simulink subsystem "AdasCorePlantModel"  (R2023a)
settings: Solver=VariableStepAuto  StartTime=0.0  StopTime=10.0  RelTol=1e-3
undefined symbols (not defined in the file or in its folder): BalNotActWait, BalOffWait, BalOnWait, Battery, contactorTime, CtrlBcuTrlrBrkGain, CtrlTcuInitGear, CtrlVcuCltch1InitCmd, CtrlVcuEvChrgLmtBpt, CtrlVcuEvRegenBrkCutOff, CtrlVcuEvRegenBrkSpdBpt, CtrlVcuEvSocBpt, currentFactor, CV_Gain, DiscIntNeverNeededParam, EnvAbsPrs, EnvAirTemp, EnvNomFrictionScaling, EnvNominalGrade, EnvWindVelX, EnvWindVelY, EnvWindVelZ, flgEnBalancing, HighTempLimit, I_cc, LowTempLimit, MaxCellVoltThrsld, MaxChrgCurrLim, MaxDchrgCurrLim, MinCellVoltDchrgCurrentLim_BP, MinCellVoltDchrgCurrentLim_Table, noCurrent, OverCellVoltageLimit, PlntBattModNumCellPar, PlntBattModNumCellSer, PlntBattNumMod, PlntBattSocInit, PlntBattTempInitDegC, PlntBrkActrBoreFrnt, PlntBrkFrntBias, PlntBrkKinFricCffFrnt, PlntBrkNumPadsFrnt, PlntBrkPadMeanRadiusFrnt, PlntBrkPrsFctr, PlntBrkRearBias, PlntDiffrntlRatio, PlntEM1EffTbl, PlntEM1Spd, PlntEM1Trq, PlntEM1TrqEff, PlntVehDstCGFrntAxl, PlntVehDstCGRearAxl, SnsrFltThld, TargetDeltaV, timeoutContactor, timeoutCurrent, Ts, UnderCellVoltageLimit, voltThreshold, vRatio
libraries: simulink x10, sharedTrackingLibrary x2, autolibutils x1
(part 3 of 4)

== system AdasCorePlantModel/Controllers/Vehicle Control Unit (VCU)/EV 1EM with BMS (non-reference)/Power Limit Calculations ==
  note: Use Current Limits from BMS to calculate
      | discharge and charge power limits
  PackVolt : Inport
  BMSDischrgCurrLmt : Inport  Port=2
  BMSChrgCurrLmt : Inport  Port=3
  Data Type Conversion : DataTypeConversion  SaturateOnIntegerOverflow=off  RndMeth=Floor
  Data Type Conversion1 : DataTypeConversion  SaturateOnIntegerOverflow=off  RndMeth=Floor
  Gain : Gain  Gain=-1
  Gain1 : Gain  Gain=-1
  Product : Product
  Product1 : Product
  BattPwrDischrgLmt : Outport  VectorParamsAs1DForOutWhenUnconnected=off
  BattPwrChrgLmt : Outport  Port=2  VectorParamsAs1DForOutWhenUnconnected=off
  wires:
  Data Type Conversion1/1 -> BattPwrDischrgLmt/1
  Data Type Conversion/1 -> BattPwrChrgLmt/1
  BMSDischrgCurrLmt/1 -> Gain1/1
  BMSChrgCurrLmt/1 -> Gain/1
  PackVolt/1 -> Product1/1, Product/1
  Product1/1 -> Data Type Conversion/1
  Product/1 -> Data Type Conversion1/1
  Gain1/1 -> Product/2
  Gain/1 -> Product1/2

== system AdasCorePlantModel/Controllers/Vehicle Control Unit (VCU)/EV 1EM with BMS (non-reference)/Regen Braking Control ==
  "BattSoc " : Inport
  "VehSpd " : Inport  Port=2
  "EMSpd " : Inport  Port=3
  "BrkPrsReq " : Inport  Port=4
  Parallel Regen Braking : Subsystem  InitFcn=[~]=autosharedicon('autolibinternalvvblock',gcb,0,'6');  VariantControl=(default)
  Series Regen Braking : Subsystem  InitFcn=%[~]=autosharedicon('autolibinternalvvblock',gcb,0,'6');  VariantControl=Variant
  " EMTrqCmdRegen" : Outport  VectorParamsAs1DForOutWhenUnconnected=off
  " BrkCmd" : Outport  Port=2  VectorParamsAs1DForOutWhenUnconnected=off

== system AdasCorePlantModel/Controllers/Vehicle Control Unit (VCU)/EV 1EM with BMS (non-reference)/Subsystem2 ==
  SOC : Inport
  Data Type Conversion : DataTypeConversion  SaturateOnIntegerOverflow=off  RndMeth=Floor
  convert2percent : Gain  Gain=100
  BattSOC : Outport
  wires:
  Data Type Conversion/1 -> BattSOC/1
  SOC/1 -> convert2percent/1
  convert2percent/1 -> Data Type Conversion/1

== system AdasCorePlantModel/Controllers/Vehicle Control Unit (VCU)/EV 1EM with BMS (non-reference)/Trailer Brake Pressure Command ==
  BrkCmd : Inport
  Gain1 : Gain  Gain=CtrlBcuTrlrBrkGain
  Probe : Probe  ProbeSampleTime=off  ProbeComplexSignal=off
  Product : Product  Inputs=*/
  Selector2 : Selector  InputPortWidth=1  IndexOptions=Index vector (dialog)  Indices=[1 1 1 1 1 1]  OutputSizes=1
  Sum : Sum  Inputs=+
  VcuTrlrBrkPrsCmd : Outport
  wires:
  Selector2/1 -> VcuTrlrBrkPrsCmd/1
  Sum/1 -> Product/1
  BrkCmd/1 -> Sum/1, Probe/1
  Probe/1 -> Product/2
  Product/1 -> Gain1/1
  Gain1/1 -> Selector2/1

== system AdasCorePlantModel/Environment/Varying Friction/Varying Friction/Road Track Friction ==
  XWhl : Inport
  YWhl : Inport  Port=2
  Cg : Inport  Port=3
  2D Lookup Tbl for Scaling Fctr (Lambda) : Subsystem  TreatAsAtomicUnit=on
      mask init:
      | [~]=vehdynicon('vehdynblk',gcb);
  Bus Selector : BusSelector  OutputSignals=X,Y
  Cnst Lambda : Constant  Value=ones(4,1).*lambda_g
  Constant1 : Constant  Value=SplitLambdaTrck
  Creating Inertial Frm Bpt : Subsystem
  En at t = 0 : Subsystem
  "Lambda (t = 0) " : Memory  InitialCondition=ones(4,1).*lambda_g  InheritSampleTime=on
  Switch : Switch  Criteria=u2 > Threshold  SaturateOnIntegerOverflow=off  InputSameDT=off
  FricCoeffLambda : Outport
  wires:
  YWhl/1 -> 2D Lookup Tbl for Scaling Fctr (Lambda)/2(YWhl)
  XWhl/1 -> 2D Lookup Tbl for Scaling Fctr (Lambda)/1(XWhl)
  2D Lookup Tbl for Scaling Fctr (Lambda)/1(Lambda for each whl) -> Switch/1
  "Lambda (t = 0) "/1 -> FricCoeffLambda/1
  Switch/1 -> "Lambda (t = 0) "/1
  Cnst Lambda/1 -> Switch/3
  Constant1/1 -> Switch/2
  Cg/1 -> Bus Selector/1
  Creating Inertial Frm Bpt/1(XBpt) -> 2D Lookup Tbl for Scaling Fctr (Lambda)/3(XBpt)
  Creating Inertial Frm Bpt/2(YBpt) -> 2D Lookup Tbl for Scaling Fctr (Lambda)/4(YBpt)
  Bus Selector/1 -> Creating Inertial Frm Bpt/1(XCg)  "<X>"
  Bus Selector/2 -> Creating Inertial Frm Bpt/2(YCg)  "<Y>"
  En at t = 0/1(Out1) -> Creating Inertial Frm Bpt/Enable

== system AdasCorePlantModel/Environment/Varying Friction/Varying Friction/Wheel Coordinates ==
  FrntAxlLftX : Inport
  FrntAxlRghtX : Inport  Port=2
  RearAxlLftX : Inport  Port=3
  RearAxlRghtX : Inport  Port=4
  FrntAxlLftY : Inport  Port=5
  FrntAxlRghtY : Inport  Port=6
  RearAxlLftY : Inport  Port=7
  RearAxlRghtY : Inport  Port=8
  Matrix Concatenate : Concatenate  NumInputs=4  Mode=Multidimensional array
  Matrix Concatenate1 : Concatenate  NumInputs=4  Mode=Multidimensional array
  XWhl : Outport
  YWhl : Outport  Port=2
  wires:
  RearAxlRghtX/1 -> Matrix Concatenate/4
  Matrix Concatenate/1 -> XWhl/1
  RearAxlRghtY/1 -> Matrix Concatenate1/4
  RearAxlLftX/1 -> Matrix Concatenate/3
  RearAxlLftY/1 -> Matrix Concatenate1/3
  FrntAxlRghtX/1 -> Matrix Concatenate/2
  FrntAxlRghtY/1 -> Matrix Concatenate1/2
  FrntAxlLftY/1 -> Matrix Concatenate1/1
  FrntAxlLftX/1 -> Matrix Concatenate/1
  Matrix Concatenate1/1 -> YWhl/1

== system AdasCorePlantModel/Vehicle/Trailer Input/Ground Info Trailer/Ground Info 2 AxleTrailer ==
  Env : Inport
  Bus Selector1 : BusSelector  OutputSignals=TraGnd.z.G_FL_z,TraGnd.z.G_FR_z,TraGnd.z.G_RL_z,TraGnd.z.G_RR_z
  Bus Selector3 : BusSelector  OutputSignals=Gnd.mu.mu_FL,Gnd.mu.mu_FR,Gnd.mu.mu_RL,Gnd.mu.mu_RR
  Vector Concatenate : Concatenate  NumInputs=4
  Vector Concatenate1 : Concatenate  NumInputs=4
  Ground : Outport
  Friction : Outport  Port=2
  wires:
  Bus Selector3/4 -> Vector Concatenate/4  "<mu_RR>"
  Bus Selector3/3 -> Vector Concatenate/3  "<mu_RL>"
  Bus Selector1/1 -> Vector Concatenate1/1  "<G_FL_z>"
  Bus Selector1/2 -> Vector Concatenate1/2  "<G_FR_z>"
  Bus Selector1/3 -> Vector Concatenate1/3  "<G_RL_z>"
  Bus Selector1/4 -> Vector Concatenate1/4  "<G_RR_z>"
  Bus Selector3/2 -> Vector Concatenate/2  "<mu_FR>"
  Bus Selector3/1 -> Vector Concatenate/1  "<mu_FL>"
  Vector Concatenate/1 -> Friction/1
  Vector Concatenate1/1 -> Ground/1
  Env/1 -> Bus Selector1/1, Bus Selector3/1

== system AdasCorePlantModel/Vehicle/Trailer Input/Ground Info Trailer/Ground Info 3 AxleTrailer ==
  Env : Inport
  Bus Selector1 : BusSelector  OutputSignals=TraGnd.z.G_FL_z,TraGnd.z.G_FR_z,TraGnd.z.G_RL_z,TraGnd.z.G_RR_z,TraGnd.z.G_RL_z,TraGnd.z.G_RR_z
  Bus Selector3 : BusSelector  OutputSignals=TraGnd.mu.mu_FL,TraGnd.mu.mu_FR,TraGnd.mu.mu_RL,TraGnd.mu.mu_RR,TraGnd.mu.mu_RL,TraGnd.mu.mu_RR
  Vector Concatenate : Concatenate  NumInputs=6
  Vector Concatenate1 : Concatenate  NumInputs=6
  Ground : Outport
  Friction : Outport  Port=2
  wires:
  Env/1 -> Bus Selector3/1, Bus Selector1/1
  Vector Concatenate1/1 -> Ground/1
  Vector Concatenate/1 -> Friction/1
  Bus Selector3/1 -> Vector Concatenate/1  "<mu_FL>"
  Bus Selector3/2 -> Vector Concatenate/2  "<mu_FR>"
  Bus Selector3/3 -> Vector Concatenate/3  "<mu_RL>"
  Bus Selector3/4 -> Vector Concatenate/4  "<mu_RR>"
  Bus Selector3/5 -> Vector Concatenate/5  "<mu_RL>"
  Bus Selector3/6 -> Vector Concatenate/6  "<mu_RR>"
  Bus Selector1/1 -> Vector Concatenate1/1  "<G_FL_z>"
  Bus Selector1/2 -> Vector Concatenate1/2  "<G_FR_z>"
  Bus Selector1/3 -> Vector Concatenate1/3  "<G_RL_z>"
  Bus Selector1/4 -> Vector Concatenate1/4  "<G_RR_z>"
  Bus Selector1/5 -> Vector Concatenate1/5  "<G_RL_z>"
  Bus Selector1/6 -> Vector Concatenate1/6  "<G_RR_z>"

== system AdasCorePlantModel/Controllers/Battery Management System (BMS)/BMS (non-reference)/Subsystem1/CalculateMinMaxCells ==
  CellVoltages : Inport
  CellTemperatures : Inport  Port=2
  Bus Creator : BusCreator  Inputs=4
  MinMax : MinMax
  MinMax1 : MinMax
  MinMax2 : MinMax  Function=max
  MinMax4 : MinMax  Function=max
  MinMaxCells : Outport  SampleTime=[0.10000000000000001,0]  VectorParamsAs1DForOutWhenUnconnected=off
  wires:
  Bus Creator/1 -> MinMaxCells/1  "MinMaxCells"
  MinMax4/1 -> Bus Creator/4  "MaxCellTemp"
  MinMax1/1 -> Bus Creator/3  "MinCellTemp"
  CellVoltages/1 -> MinMax2/1, MinMax/1
  MinMax/1 -> Bus Creator/1  "MinCellVolt"
  CellTemperatures/1 -> MinMax1/1, MinMax4/1
  MinMax2/1 -> Bus Creator/2  "MaxCellVolt"

== system AdasCorePlantModel/Controllers/Battery Management System (BMS)/BMS (non-reference)/Subsystem1/ChargeCurrentLimitCalc ==
  MinMaxCells : Inport
  Bus Selector : BusSelector  OutputSignals=MaxCellVolt,MinCellTemp,MaxCellTemp
  HighTempChrgCurrentLim : Lookup_n-D  NumberOfTableDimensions=1  BreakpointsForDimension1="single([40  45  50  55 60])"  Table=single([1.0 0.8 0.5 0.3 0])  ExtrapMethod=Clip  InternalRulePriority=Speed  RndMeth=Simplest
  LowTempChrgCurrentLim : Lookup_n-D  NumberOfTableDimensions=1  BreakpointsForDimension1=single([-15 -10 -5.0 0.0 5.0 10 15.0])  Table="single([0.1 0.2  0.3 0.3 0.5 1.0 1.0])"  ExtrapMethod=Clip  InternalRulePriority=Speed  RndMeth=Simplest
  MaxCellVoltChrgCurrentLim : Lookup_n-D  NumberOfTableDimensions=1  BreakpointsForDimension1=single([3.9 4.0 4.15 4.2])  Table="single([1.0 0.8 0.3  0.3])"  ExtrapMethod=Clip  InternalRulePriority=Speed  RndMeth=Simplest
  MaxChrgCurrLim : Gain  Gain=MaxChrgCurrLim
  MinMax2 : MinMax  Inputs=3
  Np_Module : Gain  Gain=single(PlntBattModNumCellPar)
  ChargeCurrentLimit : Outport  VectorParamsAs1DForOutWhenUnconnected=off
  wires:
  Np_Module/1 -> ChargeCurrentLimit/1  "ChargeCurrentLimit"
  Bus Selector/1 -> MaxCellVoltChrgCurrentLim/1  "<MaxCellVolt>"
  MaxCellVoltChrgCurrentLim/1 -> MinMax2/1
  Bus Selector/3 -> HighTempChrgCurrentLim/1  "<MaxCellTemp>"
  Bus Selector/2 -> LowTempChrgCurrentLim/1  "<MinCellTemp>"
  MinMaxCells/1 -> Bus Selector/1
  MaxChrgCurrLim/1 -> Np_Module/1
  LowTempChrgCurrentLim/1 -> MinMax2/2
  HighTempChrgCurrentLim/1 -> MinMax2/3
  MinMax2/1 -> MaxChrgCurrLim/1

== system AdasCorePlantModel/Controllers/Battery Management System (BMS)/BMS (non-reference)/Subsystem1/DischargeCurrentLimitCalc ==
  MinMaxCells : Inport
  Bus Selector : BusSelector  OutputSignals=MinCellVolt,MinCellTemp,MaxCellTemp
  HighTempDchrgCurrentLim : Lookup_n-D  NumberOfTableDimensions=1  BreakpointsForDimension1=single([40, 45, 50, 60])  Table=single([1, 0.5, 0.3, 0])  ExtrapMethod=Clip  InternalRulePriority=Speed  RndMeth=Simplest
  LowTempDchrgCurrentLim : Lookup_n-D  NumberOfTableDimensions=1  BreakpointsForDimension1="single([-10, -5,    0,   5, 10, 15, 20])"  Table="single([0,  0.2, 0.3, 0.5, 0.75, 1, 1])"  ExtrapMethod=Clip  InternalRulePriority=Speed  RndMeth=Simplest
  MaxDchrgCurrLim : Gain  Gain=MaxDchrgCurrLim
  MinCellVoltDchrgCurrentLim : Lookup_n-D  NumberOfTableDimensions=1  DataSpecification=Lookup table object  LookupTableObject=MinCellVoltDchrgCurrentLimTable  BreakpointsForDimension1=MinCellVoltDchrgCurrentLim_BP  Table=MinCellVoltDchrgCurrentLim_Table  ExtrapMethod=Clip  InternalRulePriority=Speed  RndMeth=Simplest
  MinMax2 : MinMax  Inputs=3
  Np_Module : Gain  Gain=single(PlntBattModNumCellPar)
  DischargeCurrentLimit : Outport  VectorParamsAs1DForOutWhenUnconnected=off
  wires:
  Bus Selector/1 -> MinCellVoltDchrgCurrentLim/1  "<MinCellVolt>"
  MinCellVoltDchrgCurrentLim/1 -> MinMax2/1  "MinCellVoltDchrgCurrentLim"
  MinMaxCells/1 -> Bus Selector/1
  Np_Module/1 -> DischargeCurrentLimit/1
  LowTempDchrgCurrentLim/1 -> MinMax2/2  "LowTempDchrgCurrentLim"
  HighTempDchrgCurrentLim/1 -> MinMax2/3  "HighTempDchrgCurrentLim"
  Bus Selector/2 -> LowTempDchrgCurrentLim/1  "<MinCellTemp>"
  Bus Selector/3 -> HighTempDchrgCurrentLim/1  "<MaxCellTemp>"
  MaxDchrgCurrLim/1 -> Np_Module/1
  MinMax2/1 -> MaxDchrgCurrLim/1

== system AdasCorePlantModel/Controllers/Battery Management System (BMS)/BMS (non-reference)/Subsystem3/Coulomb Counting ==
  Curr : Inport
  Temp : Inport  Port=2
  Capacity Dependent on Temperature : Subsystem  VariantControl=Capacity Dependent on Temperature
  Constant Capacity : Subsystem  VariantControl=Constant Capacity
  SOC : Outport

== system AdasCorePlantModel/Controllers/Battery Management System (BMS)/BMS (non-reference)/Subsystem3/SOC Kalman Filters ==
  Temperature (K) : Inport
  Enable : Inport  Port=2
  PackCurrent : Inport  Port=3
  Cell_Voltage : Inport  Port=4
  No Kalman Filters : Subsystem  VariantControl=No Kalman Filters
  SOC Kalman Filters : Subsystem  InitFcn=|  VariantControl=SOC Kalman Filters
      | if ~license('test', 'identification_toolbox') 
      |   error(['Block' gcb ' Requires System Identification Toolbox']) 
      | end 
      | 
      | if ~license('test', 'control_toolbox') 
      |     error(['Block' gcb ' Requires Control System Toolbox']) 
      | end
  SOC_UKF : Outport
  SOC_EKF : Outport  Port=2

== system AdasCorePlantModel/Controllers/Vehicle Control Unit (VCU)/EV 1EM with BMS (non-reference)/Motor Torque Arbitration and Power Management/Power Management ==
  note: Power Management algorithm:
      | - Estimate Elec power based on mech power using efficiency map
      | - Check if Elec power is within battery power limits
      | - If power within limit , use motor torque command
      | - If power limit exceeded, use limited motor torque
      | - For low Mot Spd, MotPwrReq will be a small number.  Pass through torque command until Mot Spd > 2.
  BattPwrDischrgLmt : Inport
  BattPwrChrgLmt : Inport  Port=2
  EMSpd : Inport  Port=3
  EMTrqCmd : Inport  Port=4
  SOC : Inport  Port=5
  Abs : Abs  SaturateOnIntegerOverflow=off
  Check Within Limits : Subsystem
  Compare To Constant : simulink/Logic and Bit Operations/Compare To Constant  relop=<  const=2  OutDataTypeStr=boolean
  ElecToMechPwr : Product  Inputs=*/
  Mech to Elec Power Estimate : Subsystem
  MechPwrToTrq : Product  Inputs=*/
  Switch : Switch  Criteria=u2 > Threshold  SaturateOnIntegerOverflow=off  InputSameDT=off
  Switch1 : Switch  Criteria=u2 > Threshold  SaturateOnIntegerOverflow=off  InputSameDT=off
  Torque Limit : Subsystem
  div0protect - poly : autolibutils/div0protect - poly  thresh=2  ZeroCross1=off  aMode=6
  EMTrqCmdFinal : Outport  VectorParamsAs1DForOutWhenUnconnected=off
  wires:
  SOC/1 -> Torque Limit/3(SOC)
  Compare To Constant/1 -> Switch1/2
  Abs/1 -> Compare To Constant/1
  Switch1/1 -> Torque Limit/1(EMTrq)
  Check Within Limits/1(InLimit) -> Switch/2
  Switch/1 -> Switch1/3
  Check Within Limits/2(y) -> ElecToMechPwr/1
  BattPwrChrgLmt/1 -> Check Within Limits/3(lo)
  Mech to Elec Power Estimate/1(EMPwrElecReq) -> Check Within Limits/2(u)
  BattPwrDischrgLmt/1 -> Check Within Limits/1(up)
  Torque Limit/1(EMTrqCmd) -> EMTrqCmdFinal/1
  MechPwrToTrq/1 -> Switch/3
  ElecToMechPwr/1 -> MechPwrToTrq/1
  Mech to Elec Power Estimate/2(Eff2k) -> ElecToMechPwr/2
  div0protect - poly/1 -> MechPwrToTrq/2
  EMTrqCmd/1 -> Mech to Elec Power Estimate/1(EMTrqCmd), Switch1/1, Switch/1
  EMSpd/1 -> Mech to Elec Power Estimate/2(EMSpd), div0protect - poly/1, Torque Limit/2(EMSpd), Abs/1

== system AdasCorePlantModel/Controllers/Vehicle Control Unit (VCU)/EV 1EM with BMS (non-reference)/Regen Braking Control/Parallel Regen Braking ==
  VehSpd : Inport
  "EMSpd " : Inport  Port=2
  "BrkPrsReq " : Inport  Port=3
  BattSoc : Inport  Port=4
  ChrgLmt : Lookup_n-D  NumberOfTableDimensions=1  BreakpointsForDimension1=CtrlVcuEvSocBpt  Table=CtrlVcuEvChrgLmtBpt  ExtrapMethod=Clip  UseLastTableValue=on  InternalRulePriority=Speed  RndMeth=Simplest
  Gain : Gain  Gain=-1
  MaxMotorTrqVsSpd : Lookup_n-D  NumberOfTableDimensions=1  BreakpointsForDimension1=PlntEM1Spd*30/pi  Table=PlntEM1Trq  ExtrapMethod=Clip  UseLastTableValue=on  InternalRulePriority=Speed  OutDataTypeStr=Inherit: Inherit from 'Table data'  RndMeth=Simplest
  Product1 : Product
  Product3 : Product
  RegenBrakingCutoff : Lookup_n-D  NumberOfTableDimensions=1  BreakpointsForDimension1=CtrlVcuEvRegenBrkSpdBpt  Table=CtrlVcuEvRegenBrkCutOff  ExtrapMethod=Clip  UseLastTableValue=on  InternalRulePriority=Speed  RndMeth=Simplest
  rads_to_rpm : Gain  Gain=30/pi
  " EMTrqCmdRegen" : Outport  VectorParamsAs1DForOutWhenUnconnected=off
  " BrkCmd" : Outport  Port=2  VectorParamsAs1DForOutWhenUnconnected=off
  wires:
  "BrkPrsReq "/1 -> " BrkCmd"/1  "BrkPrsReq"
  "EMSpd "/1 -> rads_to_rpm/1
  rads_to_rpm/1 -> MaxMotorTrqVsSpd/1
  MaxMotorTrqVsSpd/1 -> Product3/1  "MotTrqMax"
  ChrgLmt/1 -> Product1/2
  VehSpd/1 -> RegenBrakingCutoff/1
  RegenBrakingCutoff/1 -> Product1/1
  Product1/1 -> Product3/2  "RegenFactor"
  Product3/1 -> Gain/1  "MotTrqRegen"
  BattSoc/1 -> ChrgLmt/1
  Gain/1 -> " EMTrqCmdRegen"/1

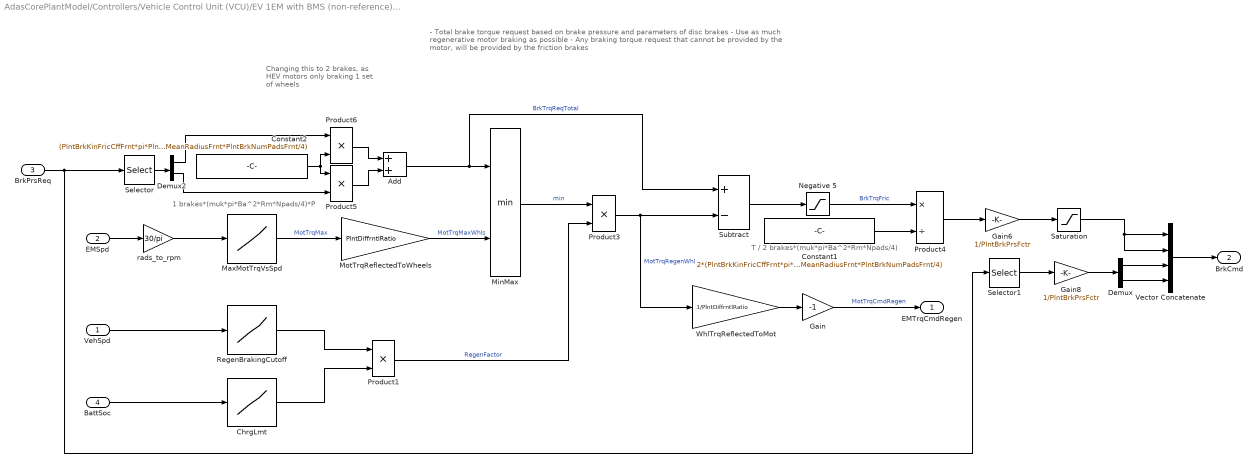
== system AdasCorePlantModel/Controllers/Vehicle Control Unit (VCU)/EV 1EM with BMS (non-reference)/Regen Braking Control/Series Regen Braking ==
  note: 1 brakes*(muk*pi*Ba^2*Rm*Npads/4)*P
  note: Changing this to 2 brakes,
      | as HEV motors only braking
      | 1 set of wheels
  note: T / 2 brakes*(muk*pi*Ba^2*Rm*Npads/4)
  note: - Total brake torque request based on brake pressure and parameters of disc brakes
      | - Use as much regenerative motor braking as possible
      | - Any braking torque request that cannot be provided by the motor, will be provided by the friction brakes
  VehSpd : Inport
  "EMSpd " : Inport  Port=2
  "BrkPrsReq " : Inport  Port=3
  BattSoc : Inport  Port=4
  Add : Sum
  ChrgLmt : Lookup_n-D  NumberOfTableDimensions=1  BreakpointsForDimension1=CtrlVcuEvSocBpt  Table=CtrlVcuEvChrgLmtBpt  ExtrapMethod=Clip  UseLastTableValue=on  InternalRulePriority=Speed  RndMeth=Simplest
  Constant1 : Constant  Value=2*(PlntBrkKinFricCffFrnt*pi*PlntBrkActrBoreFrnt^2*PlntBrkPadMeanRadiusFrnt*PlntBrkNumPadsFrnt/4)
  Constant2 : Constant  Value=(PlntBrkKinFricCffFrnt*pi*PlntBrkActrBoreFrnt^2*PlntBrkPadMeanRadiusFrnt*PlntBrkNumPadsFrnt/4)
  Demux : Demux  Outputs=2
  Demux2 : Demux  Outputs=2
  Gain : Gain  Gain=-1
  Gain6 : Gain  Gain=1/PlntBrkPrsFctr
  Gain8 : Gain  Gain=1/PlntBrkPrsFctr
  MaxMotTrqVsSpd : Lookup_n-D  NumberOfTableDimensions=1  BreakpointsForDimension1=PlntEM1Spd*30/pi  Table=PlntEM1Trq  ExtrapMethod=Clip  UseLastTableValue=on  InternalRulePriority=Speed  OutDataTypeStr=Inherit: Inherit from 'Table data'  RndMeth=Simplest
  MinMax : MinMax  Inputs=2
  MotTrqReflectedToWheels : Gain  Gain=PlntDiffrntlRatio
  Negative 5 : Saturate  UpperLimit=inf  LowerLimit=0
  Product{1,3,5..6} (4 alike) : Product
  Product4 : Product  Inputs=*/
  RegenBrakingCutoff : Lookup_n-D  NumberOfTableDimensions=1  BreakpointsForDimension1=CtrlVcuEvRegenBrkSpdBpt  Table=CtrlVcuEvRegenBrkCutOff  ExtrapMethod=Clip  UseLastTableValue=on  InternalRulePriority=Speed  RndMeth=Simplest
  Saturation : Saturate  UpperLimit=1  LowerLimit=0
  Selector : Selector  InputPortWidth=4  IndexOptions=Index vector (dialog)  Indices=[1 2]  OutputSizes=1
  Selector1 : Selector  InputPortWidth=4  IndexOptions=Index vector (dialog)  Indices=[3 4]  OutputSizes=1
  Subtract : Sum  Inputs=+-
  Vector Concatenate : Concatenate  NumInputs=4
  WhlTrqReflectedToMot : Gain  Gain=1/PlntDiffrntlRatio
  rads_to_rpm : Gain  Gain=30/pi
  " EMTrqCmdRegen" : Outport  VectorParamsAs1DForOutWhenUnconnected=off
  " BrkCmd" : Outport  Port=2  VectorParamsAs1DForOutWhenUnconnected=off
  wires:
  Demux/2 -> Vector Concatenate/4
  Product4/1 -> Gain6/1
  Demux/1 -> Vector Concatenate/3
  Gain6/1 -> Saturation/1
  Vector Concatenate/1 -> " BrkCmd"/1
  "BrkPrsReq "/1 -> Selector/1, Selector1/1
  Selector1/1 -> Gain8/1
  Saturation/1 -> Vector Concatenate/1, Vector Concatenate/2
  Gain8/1 -> Demux/1
  Add/1 -> MinMax/1, Subtract/1  "BrkTrqReqTotal"
  Product5/1 -> Add/2
  Product6/1 -> Add/1
  Selector/1 -> Demux2/1
  Demux2/1 -> Product6/1
  Constant2/1 -> Product5/1, Product6/2
  Demux2/2 -> Product5/2
  Gain/1 -> " EMTrqCmdRegen"/1  "MotTrqCmdRegen"
  WhlTrqReflectedToMot/1 -> Gain/1
  MotTrqReflectedToWheels/1 -> MinMax/2  "MotTrqMaxWhls"
  "EMSpd "/1 -> rads_to_rpm/1
  Negative 5/1 -> Product4/1  "BrkTrqFric"
  BattSoc/1 -> ChrgLmt/1
  Subtract/1 -> Negative 5/1
  Product1/1 -> Product3/2  "RegenFactor"
  RegenBrakingCutoff/1 -> Product1/1
  VehSpd/1 -> RegenBrakingCutoff/1
  ChrgLmt/1 -> Product1/2
  MinMax/1 -> Product3/1  "min"
  MaxMotTrqVsSpd/1 -> MotTrqReflectedToWheels/1  "MotTrqMax"
  rads_to_rpm/1 -> MaxMotTrqVsSpd/1
  Constant1/1 -> Product4/2
  Product3/1 -> Subtract/2, WhlTrqReflectedToMot/1  "MotTrqRegenWhl"

== system AdasCorePlantModel/Environment/Varying Friction/Varying Friction/Road Track Friction/2D Lookup Tbl for Scaling Fctr (Lambda) ==
  XWhl : Inport  Partition=on  PartitionDimension=1  PartitionWidth=1  PartitionOffset=0
  YWhl : Inport  Port=2  Partition=on  PartitionDimension=1  PartitionWidth=1  PartitionOffset=0
  XBpt : Inport  Port=3
  YBpt : Inport  Port=4
  2-D Lookup Table : Lookup_n-D  BreakpointsForDimension1Source=Input port  BreakpointsForDimension1=xbr  BreakpointsForDimension2Source=Input port  BreakpointsForDimension2=ybr  Table=mutable  ExtrapMethod=Clip  InternalRulePriority=Speed  RndMeth=Simplest
      settings: InputPortMap=u0,u1,p5,p7
  For Each : ForEach  DisableCoverage=on
  Lambda for each whl : Outport  ConcatenationDimension=1
  wires:
  XWhl/1 -> 2-D Lookup Table/1
  YWhl/1 -> 2-D Lookup Table/2
  2-D Lookup Table/1 -> Lambda for each whl/1
  XBpt/1 -> 2-D Lookup Table/3
  YBpt/1 -> 2-D Lookup Table/4

== system AdasCorePlantModel/Environment/Varying Friction/Varying Friction/Road Track Friction/Creating Inertial Frm Bpt ==
  XCg : Inport
  YCg : Inport  Port=2
  Enable : EnablePort
  Add : Sum
  Add1 : Sum
  Constant1 : Constant  Value=ybr
  Constant3 : Constant  Value=xbr
  XBpt : Outport
  YBpt : Outport  Port=2
  wires:
  Add/1 -> XBpt/1
  Constant1/1 -> Add1/1
  Add1/1 -> YBpt/1
  Constant3/1 -> Add/2
  YCg/1 -> Add1/2
  XCg/1 -> Add/1

== system AdasCorePlantModel/Environment/Varying Friction/Varying Friction/Road Track Friction/En at t = 0 ==
  Clock1 : Clock
  Compare To Zero : simulink/Logic and Bit Operations/Compare To Zero  relop===  OutDataTypeStr=boolean
  Constant : Constant
  Constant2 : Constant  Value=0
  Switch1 : Switch  Criteria=u2 > Threshold  SaturateOnIntegerOverflow=off  InputSameDT=off
  Out1 : Outport
  wires:
  Clock1/1 -> Compare To Zero/1
  Constant2/1 -> Switch1/3
  Constant/1 -> Switch1/1
  Switch1/1 -> Out1/1
  Compare To Zero/1 -> Switch1/2

== system AdasCorePlantModel/Controllers/Battery Management System (BMS)/BMS (non-reference)/Subsystem3/Coulomb Counting/Capacity Dependent on Temperature ==
  Curr : Inport
  Temp : Inport  Port=2
  1-D Lookup Table : Lookup_n-D  NumberOfTableDimensions=1  BreakpointsForDimension1=single(Battery(1).Temperature_LUT)  Table=single(Battery(1).Capacity_LUT)*PlntBattModNumCellPar  InternalRulePriority=Speed  RndMeth=Simplest
  Discrete-Time Integrator : DiscreteIntegrator  InitialCondition=single(PlntBattSocInit)  SampleTime=-1  LimitOutput=on  UpperSaturationLimit=1  LowerSaturationLimit=0  ICPrevOutput=DiscIntNeverNeededParam  ICPrevScaledInput=DiscIntNeverNeededParam
  Divide : Product  Inputs=*/
  Gain : Gain  Gain=single(1/3600)
  SOC : Outport  VectorParamsAs1DForOutWhenUnconnected=off
  wires:
  Temp/1 -> 1-D Lookup Table/1
  1-D Lookup Table/1 -> Divide/2  "Capacity"
  Divide/1 -> Discrete-Time Integrator/1
  Gain/1 -> Divide/1
  Curr/1 -> Gain/1
  Discrete-Time Integrator/1 -> SOC/1

== system AdasCorePlantModel/Controllers/Battery Management System (BMS)/BMS (non-reference)/Subsystem3/Coulomb Counting/Constant Capacity ==
  note: Capacity value should match
      | what is used in Battery Model.
      | Value obtained from Simscape
      | Battery (Table-Based) parts info
      | from a Panasonic NCR18650BD.
  Curr : Inport
  Constant : Constant  Value=single(3.153*PlntBattModNumCellPar)  SampleTime=-1
  Discrete-Time Integrator : DiscreteIntegrator  InitialCondition=single(PlntBattSocInit)  SampleTime=-1  LimitOutput=on  UpperSaturationLimit=1  LowerSaturationLimit=0  ICPrevOutput=DiscIntNeverNeededParam  ICPrevScaledInput=DiscIntNeverNeededParam
  Divide : Product  Inputs=*/
  Gain : Gain  Gain=single(1/3600)
  SOC : Outport  VectorParamsAs1DForOutWhenUnconnected=off
  wires:
  Discrete-Time Integrator/1 -> SOC/1
  Curr/1 -> Gain/1
  Gain/1 -> Divide/1
  Divide/1 -> Discrete-Time Integrator/1
  Constant/1 -> Divide/2  "Capacity"

== system AdasCorePlantModel/Controllers/Battery Management System (BMS)/BMS (non-reference)/Subsystem3/SOC Kalman Filters/No Kalman Filters ==
  Constant : Constant  Value=single(0)  SampleTime=-1
  Constant1 : Constant  Value=single(0)  SampleTime=-1
  SOC_UKF : Outport
  SOC_EKF : Outport  Port=2
  wires:
  Constant1/1 -> SOC_EKF/1  "SOC_EKF"
  Constant/1 -> SOC_UKF/1  "SOC_UKF"

== system AdasCorePlantModel/Controllers/Battery Management System (BMS)/BMS (non-reference)/Subsystem3/SOC Kalman Filters/SOC Kalman Filters ==
  Temperature (K) : Inport
  Enable : Inport  Port=2
  PackCurrent : Inport  Port=3
  Cell_Voltage : Inport  Port=4
  Compare To Constant : simulink/Logic and Bit Operations/Compare To Constant  relop=~=  const=3  OutDataTypeStr=boolean
  Measurement Function : Subsystem  TreatAsAtomicUnit=on
  State Transition Function : Subsystem  TreatAsAtomicUnit=on
  UKF_EKF_1TC : Subsystem  VariantControl=CellType==1
  SOC_UKF : Outport
  SOC_EKF : Outport  Port=2
  wires:
  Enable/1 -> Compare To Constant/1
  PackCurrent/1 -> Measurement Function/1(Current), State Transition Function/1(Current)
  UKF_EKF_1TC/1(SOC_UKF) -> SOC_UKF/1  "SOC_UKF"
  Compare To Constant/1 -> UKF_EKF_1TC/Enable
  Temperature (K)/1 -> Measurement Function/2(Temperature (K)), State Transition Function/2(Temperature K)
  UKF_EKF_1TC/2(SOC_EKF) -> SOC_EKF/1  "SOC_EKF"
  Cell_Voltage/1 -> UKF_EKF_1TC/1(Cell_Voltage)

== system AdasCorePlantModel/Controllers/Vehicle Control Unit (VCU)/EV 1EM with BMS (non-reference)/Motor Torque Arbitration and Power Management/Power Management/Check Within Limits ==
  up : Inport
  u : Inport  Port=2
  lo : Inport  Port=3
  Compare To Zero : simulink/Logic and Bit Operations/Compare To Zero  relop=>=  OutDataTypeStr=boolean
  Compare To Zero1 : simulink/Logic and Bit Operations/Compare To Zero  relop=<=  OutDataTypeStr=boolean
  Logical Operator : Logic  AllPortsSameDT=off  OutDataTypeStr=boolean
  Saturation Dynamic1 : simulink/Discontinuities/Saturation Dynamic  OutMin=[]  OutMax=[]  OutDataTypeStr=Inherit: Same as second input  OutDataType=fixdt(1, 16)  OutScaling=2^-10  DoSatur=off
  Subtract : Sum  Inputs=+-
  Subtract1 : Sum  Inputs=-+
  InLimit : Outport  VectorParamsAs1DForOutWhenUnconnected=off
  y : Outport  Port=2  VectorParamsAs1DForOutWhenUnconnected=off
  wires:
  Logical Operator/1 -> InLimit/1
  Compare To Zero1/1 -> Logical Operator/2
  Compare To Zero/1 -> Logical Operator/1
  Subtract1/1 -> Compare To Zero1/1
  Subtract/1 -> Compare To Zero/1
  u/1 -> Saturation Dynamic1/2, Subtract/2, Subtract1/1
  up/1 -> Saturation Dynamic1/1, Subtract/1
  lo/1 -> Saturation Dynamic1/3, Subtract1/2
  Saturation Dynamic1/1 -> y/1

== system AdasCorePlantModel/Controllers/Vehicle Control Unit (VCU)/EV 1EM with BMS (non-reference)/Motor Torque Arbitration and Power Management/Power Management/Mech to Elec Power Estimate ==
  note: Pelec_req = Pmech_req*Eff^k,
      | k = -1 if Motoring >= 0,
      | k = 1 if Generating < 0
  note: Using an Efficiency Map, we can estimate the
      | Electric Power from the Mechanical  Torque Request.
  note: Check if Motoring
      | or Generating
  EMTrqCmd : Inport
  EMSpd : Inport  Port=2
  Abs : Abs  SaturateOnIntegerOverflow=off
  Abs1 : Abs  SaturateOnIntegerOverflow=off
  Constant1 : Constant  Value=-1  SampleTime=-1
  Constant2 : Constant  SampleTime=-1
  Eff Map : Lookup_n-D  BreakpointsForDimension1=PlntEM1Spd*30/pi  BreakpointsForDimension2=PlntEM1TrqEff  Table=PlntEM1EffTbl  ExtrapMethod=Clip  UseLastTableValue=on  InternalRulePriority=Speed  OutDataTypeStr=Inherit: Inherit from 'Table data'  RndMeth=Simplest
      settings: InputPortMap=u0,u1
  Gain1 : Gain  Gain=1/100
  Math Function : Math  Operator=pow  SignedPower=on  OutputSignalType=real
  Product : Product
  Product3 : Product
  Product4 : Product
  Switch2 : Switch  SaturateOnIntegerOverflow=off  InputSameDT=off
  rads_to_rpm : Gain  Gain=30/pi
  EMPwrElecReq : Outport  VectorParamsAs1DForOutWhenUnconnected=off
  Eff2k : Outport  Port=2  VectorParamsAs1DForOutWhenUnconnected=off
  wires:
  EMTrqCmd/1 -> Abs1/1, Product/2, Product3/2
  EMSpd/1 -> rads_to_rpm/1, Product/1, Product3/1
  Product/1 -> Switch2/2
  rads_to_rpm/1 -> Abs/1
  Abs1/1 -> Eff Map/2
  Product4/1 -> EMPwrElecReq/1
  Math Function/1 -> Product4/2, Eff2k/1
  Gain1/1 -> Math Function/1
  Abs/1 -> Eff Map/1
  Eff Map/1 -> Gain1/1
  Constant2/1 -> Switch2/3
  Constant1/1 -> Switch2/1
  Switch2/1 -> Math Function/2
  Product3/1 -> Product4/1

== system AdasCorePlantModel/Controllers/Vehicle Control Unit (VCU)/EV 1EM with BMS (non-reference)/Motor Torque Arbitration and Power Management/Power Management/Torque Limit ==
  EMTrq : Inport
  EMSpd : Inport  Port=2
  SOC : Inport  Port=3
  Compare To Constant : simulink/Logic and Bit Operations/Compare To Constant  relop=>  const=1  OutDataTypeStr=boolean
  Constant : Constant  Value=0
  Gain : Gain  Gain=-1
  MaxEMTrqVsSpd : Lookup_n-D  NumberOfTableDimensions=1  BreakpointsForDimension1=PlntEM1Spd*30/pi  Table=PlntEM1Trq  ExtrapMethod=Clip  UseLastTableValue=on  InternalRulePriority=Speed  OutDataTypeStr=Inherit: Inherit from 'Table data'  RndMeth=Simplest
  Saturation Dynamic : simulink/Discontinuities/Saturation Dynamic  OutMin=[]  OutMax=[]  OutDataTypeStr=Inherit: Same as second input  OutDataType=fixdt(1, 16)  OutScaling=2^-10  DoSatur=off
  Switch : Switch  Criteria=u2 > Threshold  SaturateOnIntegerOverflow=off  InputSameDT=off
  rads_to_rpm : Gain  Gain=30/pi
  EMTrqCmd : Outport  VectorParamsAs1DForOutWhenUnconnected=off
  wires:
  Switch/1 -> Saturation Dynamic/1
  Constant/1 -> Switch/3
  Compare To Constant/1 -> Switch/2
  SOC/1 -> Compare To Constant/1
  Gain/1 -> Saturation Dynamic/3
  rads_to_rpm/1 -> MaxEMTrqVsSpd/1
  MaxEMTrqVsSpd/1 -> Switch/1, Gain/1
  EMSpd/1 -> rads_to_rpm/1
  Saturation Dynamic/1 -> EMTrqCmd/1
  EMTrq/1 -> Saturation Dynamic/2

== system AdasCorePlantModel/Controllers/Battery Management System (BMS)/BMS (non-reference)/Subsystem3/SOC Kalman Filters/SOC Kalman Filters/Measurement Function ==
  Current : Inport
  Temperature (K) : Inport  Port=2
  batteryMeasurementFcn : TriggerPort  TriggerType=function-call  IsSimulinkFunction=on  FunctionName=batteryMeasurementFcn  VariantControl=Variant
  Add1 : Sum  Inputs=+--
  Em Table : Lookup_n-D  BreakpointsForDimension1=Battery.SOC_LUT  BreakpointsForDimension2=Battery.Temperature_LUT  BeginIndexSearchUsingPreviousIndexResult=on  Table=Battery.Em_LUT  ExtrapMethod=Clip  InternalRulePriority=Speed  RndMeth=Simplest
      settings: InputPortMap=u0,u1
  Get SOC : Selector  InputPortWidth=2  IndexOptions=Index vector (dialog)  Indices=[1]  OutputSizes=1
  Get U1 : Selector  InputPortWidth=2  IndexOptions=Index vector (dialog)  Indices=2  OutputSizes=1
  Product : Product
  R0 Table : Lookup_n-D  BreakpointsForDimension1=Battery.SOC_LUT  BreakpointsForDimension2=Battery.Temperature_LUT  BeginIndexSearchUsingPreviousIndexResult=on  Table=Battery.R0_LUT  ExtrapMethod=Clip  InternalRulePriority=Speed  RndMeth=Simplest
      settings: InputPortMap=u0,u1
  x : ArgIn  DisableCoverage=on  OutDataTypeStr=single  PortDimensions=2  ArgumentName=x
  y : ArgOut  DisableCoverage=on  OutDataTypeStr=single  ArgumentName=y
  wires:
  x/1 -> Get U1/1, Get SOC/1
  Get SOC/1 -> R0 Table/1, Em Table/1  "SOC"
  Em Table/1 -> Add1/1
  Add1/1 -> y/1
  Temperature (K)/1 -> R0 Table/2, Em Table/2
  R0 Table/1 -> Product/1
  Current/1 -> Product/2
  Product/1 -> Add1/2
  Get U1/1 -> Add1/3  "U1"

== system AdasCorePlantModel/Controllers/Battery Management System (BMS)/BMS (non-reference)/Subsystem3/SOC Kalman Filters/SOC Kalman Filters/State Transition Function ==
  Current : Inport
  Temperature K : Inport  Port=2
  batteryStateFcn : TriggerPort  TriggerType=function-call  IsSimulinkFunction=on  FunctionName=batteryStateFcn  VariantControl=Variant
  Add : Sum
  Add1 : Sum  Inputs=-+
  C1 : Lookup_n-D  BreakpointsForDimension1=Battery.SOC_LUT  BreakpointsForDimension2=Battery.Temperature_LUT  BeginIndexSearchUsingPreviousIndexResult=on  Table=Battery.C1_LUT  ExtrapMethod=Clip  InternalRulePriority=Speed  RndMeth=Simplest
      settings: InputPortMap=u0,u1
  Constant : Constant  Value=single(Ts)  OutDataTypeStr=single
  Divide : Product  Inputs=*/
  Divide1 : Product  Inputs=*/
  Divide2 : Product  Inputs=*/
  Gain : Gain  Gain=-3600
  Get SOC : Selector  InputPortWidth=2  IndexOptions=Index vector (dialog)  Indices=1  OutputSizes=1
  Get U1 : Selector  InputPortWidth=2  IndexOptions=Index vector (dialog)  Indices=2  OutputSizes=1
  Lookup Table : Lookup_n-D  NumberOfTableDimensions=1  BreakpointsForDimension1=Battery.Temperature_LUT  BeginIndexSearchUsingPreviousIndexResult=on  Table=Battery.Capacity_LUT  InternalRulePriority=Speed  RndMeth=Simplest
  Mux : Mux  Inputs=2
  Product : Product  OutDataTypeStr=single
  Product1 : Product
  R1 : Lookup_n-D  BreakpointsForDimension1=Battery.SOC_LUT  BreakpointsForDimension2=Battery.Temperature_LUT  BeginIndexSearchUsingPreviousIndexResult=on  Table=Battery.R1_LUT  ExtrapMethod=Clip  InternalRulePriority=Speed  RndMeth=Simplest
      settings: InputPortMap=u0,u1
  x : ArgIn  DisableCoverage=on  OutDataTypeStr=single  PortDimensions=2  ArgumentName=x
  xNext : ArgOut  DisableCoverage=on  OutDataTypeStr=single  PortDimensions=2  ArgumentName=xNext
  wires:
  Mux/1 -> Product/1  "xdot"
  Add1/1 -> Mux/2  "xdot_2"
  Divide2/1 -> Add1/1
  Divide1/1 -> Add1/2  "Current/C1"
  C1/1 -> Divide1/2, Product1/2  "C1"
  R1/1 -> Product1/1  "R1"
  Product1/1 -> Divide2/2  "R1*C1"
  Get U1/1 -> Divide2/1  "U1"
  Divide/1 -> Mux/1  "xdot_1"
  Gain/1 -> Divide/2
  x/1 -> Get SOC/1, Get U1/1, Add/1
  Add/1 -> xNext/1
  Temperature K/1 -> R1/2, C1/2, Lookup Table/1
  Get SOC/1 -> R1/1, C1/1
  Current/1 -> Divide/1, Divide1/1  "Current"
  Constant/1 -> Product/2
  Product/1 -> Add/2
  Lookup Table/1 -> Gain/1  "Cq"

== system AdasCorePlantModel/Controllers/Battery Management System (BMS)/BMS (non-reference)/Subsystem3/SOC Kalman Filters/SOC Kalman Filters/UKF_EKF_1TC ==
  Cell_Voltage : Inport
  Enable : EnablePort
  EKF : sharedTrackingLibrary/Extended Kalman Filter  StateTransitionFcn=batteryStateFcn  HasStateTransitionJacobianFcn=off  HasAdditiveProcessNoise=Additive  ProcessNoise=1e-10*eye(2)  HasTimeVaryingProcessNoise=off  HasStateTransitionFcnExtraArgument=0  InitialState=[single(PlntBattSocInit+0.05); 0;]  InitialStateCovariance=[1e-5 1]  MeasurementFcn1=batteryMeasurementFcn  HasMeasurementJacobianFcn1=off  HasMeasurementEnablePort1=off  HasAdditiveMeasurementNoise1=Additive  MeasurementNoise1=1e-1  HasTimeVaryingMeasurementNoise1=off  HasMeasurementFcnExtraArgument1=0  HasMeasurementWrapping1=off  MeasurementFcn2=myMeasurementFcn  HasMeasurementJacobianFcn2=off  HasMeasurementEnablePort2=off  HasAdditiveMeasurementNoise2=Additive  MeasurementNoise2=1  HasTimeVaryingMeasurementNoise2=off  HasMeasurementFcnExtraArgument2=0  HasMeasurementWrapping2=off  MeasurementFcn3=myMeasurementFcn  HasMeasurementJacobianFcn3=off  HasMeasurementEnablePort3=off  HasAdditiveMeasurementNoise3=Additive  MeasurementNoise3=1  HasTimeVaryingMeasurementNoise3=off  HasMeasurementFcnExtraArgument3=0  HasMeasurementWrapping3=off  MeasurementFcn4=myMeasurementFcn  HasMeasurementJacobianFcn4=off  HasMeasurementEnablePort4=off  HasAdditiveMeasurementNoise4=Additive  MeasurementNoise4=1  HasTimeVaryingMeasurementNoise4=off  HasMeasurementFcnExtraArgument4=0  HasMeasurementWrapping4=off  MeasurementFcn5=myMeasurementFcn  HasMeasurementJacobianFcn5=off  HasMeasurementEnablePort5=off  HasAdditiveMeasurementNoise5=Additive  MeasurementNoise5=1  HasTimeVaryingMeasurementNoise5=off  HasMeasurementFcnExtraArgument5=0  HasMeasurementWrapping5=off  EnableMultirate=off  StateTransitionFcnSampleTime=1  MeasurementFcn1SampleTime=1  MeasurementFcn2SampleTime=1  MeasurementFcn3SampleTime=1  MeasurementFcn4SampleTime=1  MeasurementFcn5SampleTime=1  UseCurrentEstimator=on  OutputStateCovariance=off  DataType=single  SampleTime=Ts  NumberOfMeasurements=1
  SOC : Selector  InputPortWidth=2  IndexOptions=Index vector (dialog)  Indices=1  OutputSizes=1
  SOC1 : Selector  InputPortWidth=2  IndexOptions=Index vector (dialog)  Indices=1  OutputSizes=1
  UKF : sharedTrackingLibrary/Unscented Kalman Filter  StateTransitionFcn=batteryStateFcn  HasAdditiveProcessNoise=Additive  ProcessNoise=1e-10*eye(2)  HasTimeVaryingProcessNoise=off  HasStateTransitionFcnExtraArgument=0  InitialState=[single(PlntBattSocInit+0.05); 0;]  InitialStateCovariance=[1e-5 1]  Alpha=1  Beta=2  Kappa=1  MeasurementFcn1=batteryMeasurementFcn  HasMeasurementEnablePort1=off  HasAdditiveMeasurementNoise1=Additive  MeasurementNoise1=0.1  HasTimeVaryingMeasurementNoise1=off  HasMeasurementFcnExtraArgument1=0  HasMeasurementWrapping1=off  MeasurementFcn2=myMeasurementFcn  HasMeasurementEnablePort2=off  HasAdditiveMeasurementNoise2=Additive  MeasurementNoise2=1  HasTimeVaryingMeasurementNoise2=off  HasMeasurementFcnExtraArgument2=0  HasMeasurementWrapping2=off  MeasurementFcn3=myMeasurementFcn  HasMeasurementEnablePort3=off  HasAdditiveMeasurementNoise3=Additive  MeasurementNoise3=1  HasTimeVaryingMeasurementNoise3=off  HasMeasurementFcnExtraArgument3=0  HasMeasurementWrapping3=off  MeasurementFcn4=myMeasurementFcn  HasMeasurementEnablePort4=off  HasAdditiveMeasurementNoise4=Additive  MeasurementNoise4=1  HasTimeVaryingMeasurementNoise4=off  HasMeasurementFcnExtraArgument4=0  HasMeasurementWrapping4=off  MeasurementFcn5=myMeasurementFcn  HasMeasurementEnablePort5=off  HasAdditiveMeasurementNoise5=Additive  MeasurementNoise5=1  HasTimeVaryingMeasurementNoise5=off  HasMeasurementFcnExtraArgument5=0  HasMeasurementWrapping5=off  EnableMultirate=off  StateTransitionFcnSampleTime=-1  MeasurementFcn1SampleTime=-1  MeasurementFcn2SampleTime=-1  MeasurementFcn3SampleTime=-1  MeasurementFcn4SampleTime=-1  MeasurementFcn5SampleTime=-1  UseCurrentEstimator=on  OutputStateCovariance=off  DataType=single  SampleTime=Ts  NumberOfMeasurements=1
  SOC_UKF : Outport  VectorParamsAs1DForOutWhenUnconnected=off
  SOC_EKF : Outport  Port=2  VectorParamsAs1DForOutWhenUnconnected=off
  wires:
  SOC/1 -> SOC_EKF/1  "SOC_EKF"
  EKF/1 -> SOC/1
  SOC1/1 -> SOC_UKF/1  "SOC_UKF"
  Cell_Voltage/1 -> EKF/1, UKF/1
  UKF/1 -> SOC1/1

== stateflow chart AdasCorePlantModel/Controllers/Battery Management System (BMS)/BMS (non-reference)/Subsystem/Balancing ==
  state BalancingOFF
    en:
    BalCmd(:,:) = false;
    en,du:
    DeltaCellVolt = MaxCellVolt - MinCellVolt;
  state BalancingON
    en, du:
    DeltaCellVolt = MaxCellVolt - MinCellVolt;
    state BalActive
      en, du:
      BalCmd = ((CellVoltages - MinCellVolt) > TargetDeltaV/2)';
      flgBalCompl = all(~BalCmd);
    state BalNotActive
    (default) -> BalActive
    BalNotActive -> BalActive [order 1] : [after(BalNotActWait,sec) && ...
        | DeltaCellVolt > TargetDeltaV]
    BalActive -> BalNotActive : [flgBalCompl]
  (default) -> BalancingOFF : {flgBalCompl = true;}
  BalancingOFF -> BalancingON : [flgEnBalancing && ...
      | BMS_State ~= 2 && ...
      | after(BalOffWait,sec) && ...
      | DeltaCellVolt > TargetDeltaV]
  BalancingON -> BalancingOFF : [BMS_State == 2]
      | %In Driving State
  BalNotActive -> BalancingOFF [order 2] : [after(BalOnWait,sec)]
  data: BMS_State input; CellVoltages input single; TargetDeltaV parameter; BalCmd output boolean size=[1,PlntBattModNumCellSer*PlntBattNumMod] =boolean(zeros(1,PlntBattModNumCellSer*PlntBattNumMod)); flgBalCompl local; MaxCellVolt input single; MinCellVolt input single; BalNotActWait parameter; BalOffWait parameter; BalOnWait parameter; flgEnBalancing parameter; DeltaCellVolt local single =single(0)
